simulink model "lab3_08_sine_compare"  (R2025b)
settings: Solver=ode45  StartTime=0.0  StopTime=30.0  MaxStep=0.01  RelTol=1e-6
settings Model: Creator=Boris  LastModifiedBy=Boris

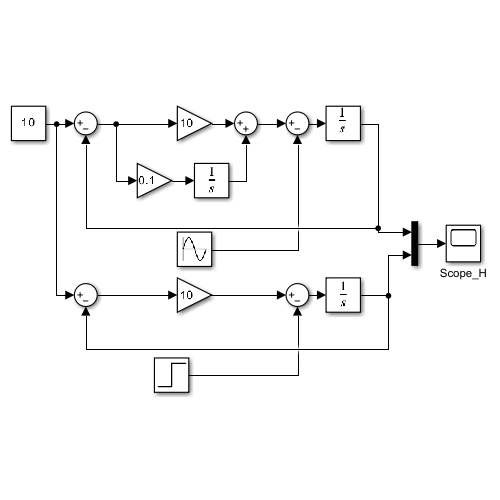
[thumbnail: Simulink's stored preview of the top-level diagram]
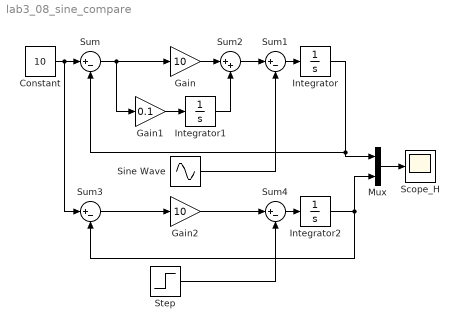
== system lab3_08_sine_compare ==
  Constant : Constant  Value=10
  Gain : Gain  Gain=10
  Gain1 : Gain  Gain=0.1
  Gain2 : Gain  Gain=10
  Integrator : Integrator
  Integrator1 : Integrator
  Integrator2 : Integrator
  Mux : Mux  Inputs=2
  Scope_H : Scope
      settings: ActiveDisplayYMinimum=-12.737485297214677  ActiveDisplayYMaximum=18.6045938448039
  Sine Wave : Sin  Amplitude=4  Frequency=2  SampleTime=0
  Step : Step  Time=6  After=2  SampleTime=0
  Sum{,1,3..4} (4 alike) : Sum  Inputs=|+-
  Sum2 : Sum  Inputs=|++
  wires:
  Integrator/1 -> Mux/1, Sum/2
  Sum/1 -> Gain1/1, Gain/1
  Gain1/1 -> Integrator1/1
  Sum1/1 -> Integrator/1
  Gain/1 -> Sum2/1
  Sum2/1 -> Sum1/1
  Integrator1/1 -> Sum2/2
  Sine Wave/1 -> Sum1/2
  Sum3/1 -> Gain2/1
  Constant/1 -> Sum3/1, Sum/1
  Integrator2/1 -> Mux/2, Sum3/2
  Gain2/1 -> Sum4/1
  Step/1 -> Sum4/2
  Sum4/1 -> Integrator2/1
  Mux/1 -> Scope_H/1
